simulink model "MRACDireto_Trab1_Regra_MIT_Pedro"  (R2015a)
settings: Solver=ode1  StartTime=0.0  StopTime=10  FixedStep=1e-3  RelTol=1e-3
undefined symbols (not defined in the file): b, gamma, it, ref, theta_c_ini
libraries: simulink x3
settings Model: Creator=user  LastModifiedBy=user

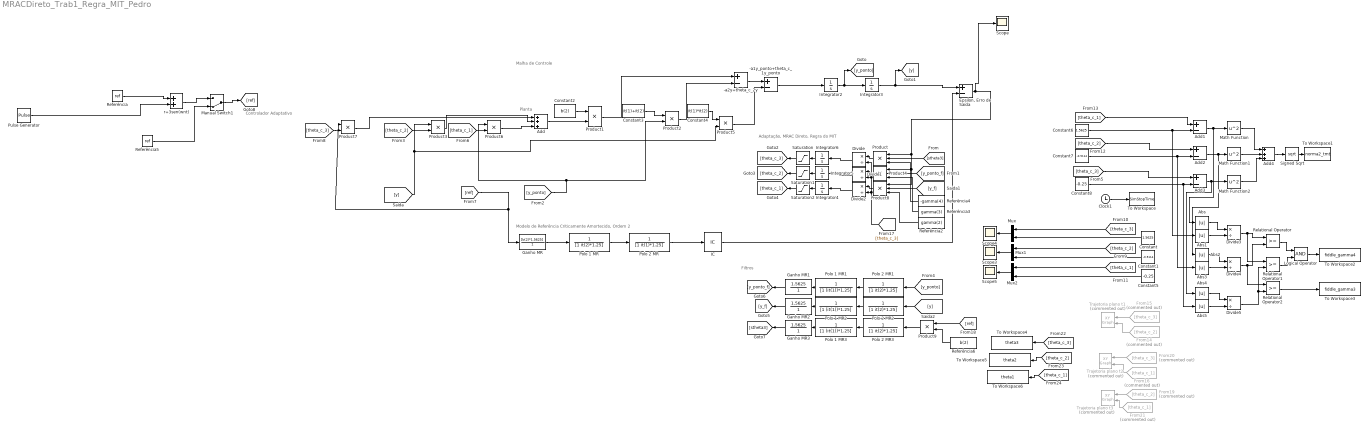
== system MRACDireto_Trab1_Regra_MIT_Pedro ==
  note: Filtros
  note: Planta
  note: Malha de Controle
  note: Modelo de Referência Criticamente Amortecido, Ordem 2
  note: Controlador Adaptativo
  note: Adaptação, MRAC Direto, Regra do MIT
  "  Referência" : Constant  Value=ref
  "  Referência2" : Constant  Value=gamma(2)
  "  Referência3" : Constant  Value=gamma(3)
  "  Referência4" : Constant  Value=-gamma(4)
  "  Referência5" : Constant  Value=ref
  "  Referência6" : Constant  Value=b(2)
  -a1y_ponto+theta_c_1y_ponto : Sum  Inputs=+-
  -a2y+theta_c_2y : Sum  Inputs=+-
  Abs{,1..5} (6 alike) : Abs
  Add : Sum  Inputs=+++
  Add1 : Sum  Inputs=+-
  Add2 : Sum  Inputs=+-
  Add3 : Sum  Inputs=+-
  Add4 : Sum  Inputs=+++
  Clock1 : Clock
  Constant : Constant  Value=1.5625
  Constant1 : Constant  Value=-0.5114
  Constant2 : Constant  Value=b(2)
  Constant3 : Constant  Value=it(1)+it(2)
  Constant4 : Constant  Value=it(1)*it(2)
  Constant5 : Constant  Value=-0.25
  Constant6 : Constant  Value=1.5625
  Constant7 : Constant  Value=-0.5114
  Constant8 : Constant  Value=-0.25
  Divide{,1..5} (6 alike) : Product  Inputs=*/
  "Epsilon, Erro de Saída" : Sum  Inputs=+-
  From14 : From  Commented=on  GotoTag=theta_c_2
  From15 : From  Commented=on  GotoTag=theta_c_3
  From16 : From  Commented=on  GotoTag=theta_c_1
  From19 : From  Commented=on  GotoTag=theta_c_2
  From20 : From  Commented=on  GotoTag=theta_c_3
  From21 : From  Commented=on  GotoTag=theta_c_1
  Ganho MR : TransferFcn  Numerator=[b(2)*1.5625]  Denominator=[1]
  Ganho MR1 : TransferFcn  Numerator=[1.5625]  Denominator=[1]
  Ganho MR2 : TransferFcn  Numerator=[1.5625]  Denominator=[1]
  Ganho MR3 : TransferFcn  Numerator=[1.5625]  Denominator=[1]
  IC : InitialCondition  Value=2
  Integrator2 : Integrator
  Integrator3 : Integrator  InitialCondition=3
  Integrator4 : Integrator  InitialCondition=theta_c_ini(4)
  Integrator5 : Integrator  InitialCondition=theta_c_ini(3)
  Integrator6 : Integrator  InitialCondition=theta_c_ini(2)
  Logical Operator : Logic  AllPortsSameDT=off  OutDataTypeStr=boolean
  Manual Switch1 : ManualSwitch  CurrentSetting=0
  Math Function : Math  Operator=square  SaturateOnIntegerOverflow=on
  Math Function1 : Math  Operator=square  SaturateOnIntegerOverflow=on
  Math Function2 : Math  Operator=square  SaturateOnIntegerOverflow=on
  Mux : Mux  Inputs=2
  Mux1 : Mux  Inputs=2
  Mux2 : Mux  Inputs=2
  Polo 1 MR : TransferFcn  Denominator=[1 it(2)*1.25]
  Polo 1 MR1 : TransferFcn  Denominator=[1 (it(1))*1.25]
  Polo 1 MR2 : TransferFcn  Denominator=[1 (it(1))*1.25]
  Polo 1 MR3 : TransferFcn  Denominator=[1 (it(1))*1.25]
  Polo 2 MR : TransferFcn  Denominator=[1 it(1)*1.25]
  Polo 2 MR1 : TransferFcn  Denominator=[1 it(2)*1.25]
  Polo 2 MR2 : TransferFcn  Denominator=[1 it(2)*1.25]
  Polo 2 MR3 : TransferFcn  Denominator=[1 it(2)*1.25]
  Product : Product  Inputs=3
  Product{1..3,5..7,9} (7 alike) : Product
  Product4 : Product  Inputs=3
  Product8 : Product  Inputs=3
  Pulse Generator : DiscretePulseGenerator  PulseType=Time based  Amplitude=0.1  Period=1  PulseWidth=50
  Relational Operator : RelationalOperator  OutDataTypeStr=boolean
  Relational Operator1 : RelationalOperator  OutDataTypeStr=boolean
  Relational Operator2 : RelationalOperator  OutDataTypeStr=boolean
  Saturation : Saturate  UpperLimit=2  LowerLimit=0
  Saturation1 : Saturate  UpperLimit=0  LowerLimit=-1
  Saturation2 : Saturate  UpperLimit=0  LowerLimit=-1
  Scope{,3..5} (4 alike) : Scope
      Scope settings: TimeRange=200  YMin=-1.51545e-14  YMax=-1.37113e-14
      Scope3 settings: TimeRange=60  YMin=-0.52  YMax=-0.42  SaveName=ScopeData3
      Scope4 settings: TimeRange=60  YMin=1.47  YMax=1.57  SaveName=ScopeData4
      Scope5 settings: YMin=-0.25  YMax=-0.2  SaveName=ScopeData5
  Signed Sqrt : Sqrt  SaturateOnIntegerOverflow=on
  To Workspace : ToWorkspace  VariableName=SimStopTime  SaveFormat=Timeseries  SampleTime=-1
  To Workspace1 : ToWorkspace  VariableName=norma2_tmt  SampleTime=-1
      settings: MaxDataPoints=1
  To Workspace2 : ToWorkspace  VariableName=fiddle_gamma4  SampleTime=-1
      settings: MaxDataPoints=1
  To Workspace3 : ToWorkspace  VariableName=fiddle_gamma3  SampleTime=-1
      settings: MaxDataPoints=1
  To Workspace4 : ToWorkspace  VariableName=theta3  SampleTime=-1
  To Workspace5 : ToWorkspace  VariableName=theta2  SampleTime=-1
  To Workspace6 : ToWorkspace  VariableName=theta1  SampleTime=-1
  Trajetoria plano t1 : simulink/Sinks/XY Graph  Commented=on  xmin=1  xmax=1.8  ymin=-0.6  ymax=-0.1  st=-1
  Trajetoria plano t2 : simulink/Sinks/XY Graph  Commented=on  xmin=1  xmax=1.8  ymin=-0.6  ymax=-0.1  st=-1
  Trajetoria plano t3 : simulink/Sinks/XY Graph  Commented=on  xmin=-0.6  xmax=0  ymin=-0.6  ymax=-0.1  st=-1
  r+3sen(wnt) : Sum
  wires:
  Ganho MR/1 -> Polo 1 MR/1
  Polo 1 MR/1 -> Polo 2 MR/1
  Polo 2 MR/1 -> IC/1
  Integrator3/1 -> [y], "Epsilon, Erro de Saída"/1
  Integrator2/1 -> [y_ponto], Integrator3/1
  -a1y_ponto+theta_c_1y_ponto/1 -> Integrator2/1
  -a2y+theta_c_2y/1 -> -a1y_ponto+theta_c_1y_ponto/1
  Product2/1 -> -a2y+theta_c_2y/2
  Constant3/1 -> Product2/1
  Product1/1 -> -a2y+theta_c_2y/1
  [y] -> Product5/2, Product3/1
  [theta_c_2] -> Product3/2
  Constant4/1 -> Product5/1
  [y_ponto] -> Product2/2, Product6/1
  [theta_c_1] -> Product6/2
  Product5/1 -> -a1y_ponto+theta_c_1y_ponto/2
  Constant2/1 -> Product1/1
  [theta_c_3] -> Product7/2
  [stheta3] -> Product/2
  [y_ponto_f] -> Product4/2
  [y_f] -> Product8/2
  "  Referência4"/1 -> Product/3
  "  Referência3"/1 -> Product4/3
  "  Referência2"/1 -> Product8/3
  Polo 2 MR1/1 -> Polo 1 MR1/1
  Polo 1 MR1/1 -> Ganho MR1/1
  [y_ponto] -> Polo 2 MR1/1
  Polo 2 MR2/1 -> Polo 1 MR2/1
  Polo 1 MR2/1 -> Ganho MR2/1
  [y] -> Polo 2 MR2/1
  Ganho MR1/1 -> [y_ponto_f]
  Ganho MR2/1 -> [y_f]
  Polo 2 MR3/1 -> Polo 1 MR3/1
  Polo 1 MR3/1 -> Ganho MR3/1
  Product9/1 -> Polo 2 MR3/1
  Ganho MR3/1 -> [stheta3]
  [ref] -> Ganho MR/1, Product7/1
  "  Referência"/1 -> r+3sen(wnt)/1
  "Epsilon, Erro de Saída"/1 -> Scope/1, Product8/1, Product4/1, Product/1
  Manual Switch1/1 -> [ref]
  r+3sen(wnt)/1 -> Manual Switch1/1
  "  Referência5"/1 -> Manual Switch1/2
  Clock1/1 -> To Workspace/1
  Product7/1 -> Add/1
  Product3/1 -> Add/2
  Product6/1 -> Add/3
  Add/1 -> Product1/2
  Pulse Generator/1 -> r+3sen(wnt)/2
  Integrator6/1 -> Saturation/1
  Integrator5/1 -> Saturation1/1
  Integrator4/1 -> Saturation2/1
  Product/1 -> Divide/1
  Product4/1 -> Divide1/1
  Product8/1 -> Divide2/1
  [theta_c_3] -> Divide2/2, Divide1/2, Divide/2
  Divide2/1 -> Integrator4/1
  Divide1/1 -> Integrator5/1
  Divide/1 -> Integrator6/1
  [ref] -> Product9/1
  "  Referência6"/1 -> Product9/2
  Mux/1 -> Scope4/1
  Mux1/1 -> Scope3/1
  Mux2/1 -> Scope5/1
  [theta_c_1] -> Mux2/1
  [theta_c_2] -> Mux1/1
  [theta_c_3] -> Mux/1
  Constant/1 -> Mux/2
  Constant1/1 -> Mux1/2
  Constant5/1 -> Mux2/2
  [theta_c_1] -> Add1/1
  [theta_c_2] -> Add2/1
  [theta_c_3] -> Add3/1
  Constant6/1 -> Abs1/1, Add1/2
  Constant7/1 -> Abs3/1, Add2/2
  Constant8/1 -> Abs5/1, Add3/2
  Add1/1 -> Abs/1, Math Function/1
  Add2/1 -> Abs2/1, Math Function1/1
  Add3/1 -> Abs4/1, Math Function2/1
  Math Function/1 -> Add4/1
  Math Function1/1 -> Add4/2
  Math Function2/1 -> Add4/3
  Add4/1 -> Signed Sqrt/1
  Signed Sqrt/1 -> To Workspace1/1
  Relational Operator/1 -> Logical Operator/1
  Relational Operator1/1 -> Logical Operator/2
  Logical Operator/1 -> To Workspace2/1
  Relational Operator2/1 -> To Workspace3/1
  Abs1/1 -> Divide3/2
  Abs/1 -> Divide3/1
  Abs3/1 -> Divide4/2
  Abs2/1 -> Divide4/1
  Abs5/1 -> Divide5/2
  Abs4/1 -> Divide5/1
  Divide3/1 -> Relational Operator1/1, Relational Operator/1
  Divide4/1 -> Relational Operator2/1, Relational Operator/2
  Divide5/1 -> Relational Operator2/2, Relational Operator1/2
  From15/1 -> Trajetoria plano t1/1
  From14/1 -> Trajetoria plano t1/2
  From20/1 -> Trajetoria plano t2/1
  From16/1 -> Trajetoria plano t2/2
  From19/1 -> Trajetoria plano t3/1
  From21/1 -> Trajetoria plano t3/2
  [theta_c_3] -> To Workspace4/1
  [theta_c_2] -> To Workspace5/1
  [theta_c_1] -> To Workspace6/1
  Saturation/1 -> [theta_c_3]
  Saturation1/1 -> [theta_c_2]
  Saturation2/1 -> [theta_c_1]
  IC/1 -> "Epsilon, Erro de Saída"/2
